simulink model "models"  (R2017a)
settings: Solver=VariableStepAuto  StartTime=0.0  StopTime=250  RelTol=1e-3
values from neighbouring files (symbols this model uses):
  k1 = 67/90    (= 0.744444444444)    [step.m]
  k2 = (93.58-64.36)/(107-90)    (= 1.71882352941)    [step.m]
  k3 = 93.13/107    (= 0.870373831776)    [step.m]
  tau1 = 34.7-33.8    (= 0.9)    [step.m]
  tau2 = 64.78-64.36    (= 0.42)    [step.m]
  tau3 = 127.1-126.8    (= 0.3)    [step.m]
settings Model: Creator=user  LastModifiedBy=user

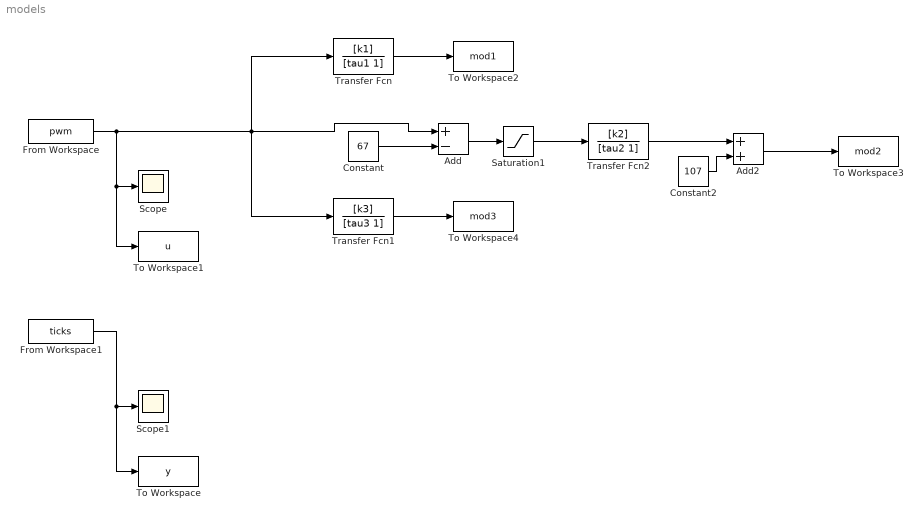
== system models ==
  Add : Sum  Inputs=+-
  Add2 : Sum
  Constant : Constant  Value=67
  Constant2 : Constant  Value=107
  From Workspace : FromWorkspace  VariableName=pwm  SampleTime=0  Interpolate=off  OutputAfterFinalValue=Holding final value
  From Workspace1 : FromWorkspace  VariableName=ticks  SampleTime=0  Interpolate=off  OutputAfterFinalValue=Holding final value
  Saturation1 : Saturate  UpperLimit=400  LowerLimit=0
  Scope : Scope
  Scope1 : Scope
  To Workspace : ToWorkspace  VariableName=y  SaveFormat=Timeseries  SampleTime=-1
  To Workspace1 : ToWorkspace  VariableName=u  SaveFormat=Timeseries  SampleTime=-1
  To Workspace2 : ToWorkspace  VariableName=mod1  SaveFormat=Timeseries  SampleTime=-1
  To Workspace3 : ToWorkspace  VariableName=mod2  SaveFormat=Timeseries  SampleTime=-1
  To Workspace4 : ToWorkspace  VariableName=mod3  SaveFormat=Timeseries  SampleTime=-1
  Transfer Fcn : TransferFcn  Numerator=[k1]  Denominator=[tau1 1]
  Transfer Fcn1 : TransferFcn  Numerator=[k3]  Denominator=[tau3 1]
  Transfer Fcn2 : TransferFcn  Numerator=[k2]  Denominator=[tau2 1]
  wires:
  From Workspace/1 -> Add/1, Transfer Fcn/1, Transfer Fcn1/1, To Workspace1/1, Scope/1
  From Workspace1/1 -> Scope1/1, To Workspace/1
  Transfer Fcn/1 -> To Workspace2/1
  Transfer Fcn1/1 -> To Workspace4/1
  Constant/1 -> Add/2
  Constant2/1 -> Add2/2
  Transfer Fcn2/1 -> Add2/1
  Add2/1 -> To Workspace3/1
  Add/1 -> Saturation1/1
  Saturation1/1 -> Transfer Fcn2/1
